simulink model "simulink_model_closed_loop"  (R2025b)
settings: Solver=daessc  StartTime=0.0  StopTime=10  RelTol=1e-3
values from neighbouring files (symbols this model uses):
  N = 40    [minimal_example_ocp.m]    (also in ocp_cart_pole.m = 20)
  nu = length(model.u)    [minimal_example_ocp.m]    (also in ocp_cart_pole.m)
  ny_0 = nu    [minimal_example_ocp.m]    (also in ocp_cart_pole.m)
  T = 1    [minimal_example_ocp.m]    (also in ocp_cart_pole.m)
undefined symbols (not defined in the file or in its folder): X, Y, Z
libraries: sm_lib x40, nesl_utility x19
(part 2 of 2)

== matlab function simulink_model_closed_loop/MATLAB Function ==
  data: ang input; ang_wrapped output
function ang_wrapped = wrapTo2PiCustom(ang)
% wrapTo2PiCustom Envuelve ángulos al rango [0, 2*pi)
%
%   ang_wrapped = wrapTo2PiCustom(ang)
%
%   ang puede ser escalar, vector o matriz (en radianes)

    ang_wrapped = mod(ang, 2*pi);

    % Asegura que 2*pi no aparezca (opcional, por consistencia matemática)
    ang_wrapped(ang_wrapped == 2*pi) = 0;
end
